simulink library "SHLA_lib"  (Simulink 7.5)
settings: Solver=ode45  StartTime=0.0  StopTime=10.0  RelTol=1e-3
values from neighbouring files (symbols this model uses):
  p_SHLA_LockPVehSpdThd_kmph = Simulink.Parameter    [SHLA_FAW_par.m]
  p_SHLA_SmplCyc_s = Simulink.Parameter    [SHLA_FAW_par.m]
  p_SHLA_TiDlyShiftLvr_s = Simulink.Parameter    [SHLA_FAW_par.m]
  p_SHLA_VehSpdThd_kmph = Simulink.Parameter    [SHLA_FAW_par.m]
  pEpark_st_Parked_C = Simulink.Parameter    [SHLA_FAW_par.m]
  pEpark_st_ParkFlt_C = Simulink.Parameter    [SHLA_FAW_par.m]
  pEpark_st_Parking_C = Simulink.Parameter    [SHLA_FAW_par.m]
  pEpark_st_ParkLocked_C = Simulink.Parameter    [SHLA_FAW_par.m]
  pEpark_st_ParkLockUnknown_C = Simulink.Parameter    [SHLA_FAW_par.m]
  pEpark_st_ParkReq_C = Simulink.Parameter    [SHLA_FAW_par.m]
  pEpark_st_ParkReqOff_C = Simulink.Parameter    [SHLA_FAW_par.m]
  pEpark_st_ParkStalled_C = Simulink.Parameter    [SHLA_FAW_par.m]
  pEpark_st_ParkUnlocked_C = Simulink.Parameter    [SHLA_FAW_par.m]
  pEpark_st_Unparked_C = Simulink.Parameter    [SHLA_FAW_par.m]
  pEpark_st_UnparkedStalled_C = Simulink.Parameter    [SHLA_FAW_par.m]
  pEpark_st_Unparking_C = Simulink.Parameter    [SHLA_FAW_par.m]
  pEpark_st_UnParkReq_C = Simulink.Parameter    [SHLA_FAW_par.m]
  pSHLA_s_StalledDelyTime_C = Simulink.Parameter    [SHLA_FAW_par.m]
undefined symbols (not defined in the file or in its folder): DiscIntNeverNeededParam, p_bool_False_M, p_bool_True_M, pMCI_rpm_VehMoveSpdThrsh_C, pMCI_rpm_VehStdStlSpdThrsh_C, pMCI_s_VehStdStlDly_C, PrkgLockStsTyp, pSHLI_bool_EparkStEnbl, ShiftLvrPosnICTyp, ShiftLvrPosnTyp
libraries: BaseOperationLib_Browser x49, PES_CZ_FAW x2, simulink x2
settings Model: Creator=wuaibin  LastModifiedBy=wuaibin

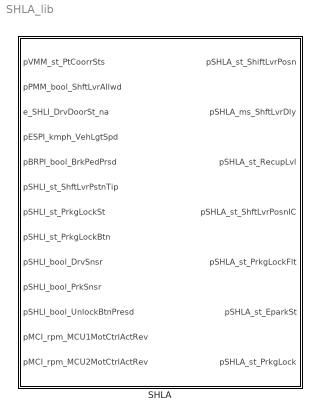
== system SHLA_lib ==
  SHLA : Subsystem  TreatAsAtomicUnit=on

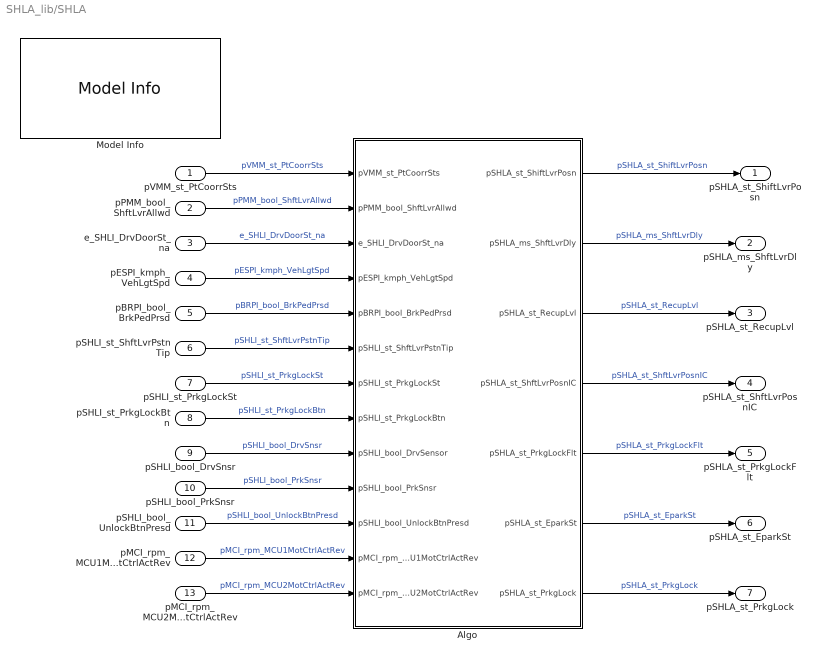
== system SHLA_lib/SHLA ==
  pVMM_st_PtCoorrSts : Inport  OutDataType=fixdt(1, 16)  OutScaling=2^0
  pPMM_bool_ShftLvrAllwd : Inport  Port=2  OutDataType=fixdt(1, 16)  OutScaling=2^0
  e_SHLI_DrvDoorSt_na : Inport  Port=3  OutDataType=fixdt(1, 16)  OutScaling=2^0
  pESPI_kmph_VehLgtSpd : Inport  Port=4  OutDataType=fixdt(1, 16)  OutScaling=2^0
  pBRPI_bool_BrkPedPrsd : Inport  Port=5  OutDataType=fixdt(1, 16)  OutScaling=2^0
  pSHLI_st_ShftLvrPstnTip : Inport  Port=6  OutDataType=fixdt(1, 16)  OutScaling=2^0
  pSHLI_st_PrkgLockSt : Inport  Port=7  OutDataType=fixdt(1, 16)  OutScaling=2^0
  pSHLI_st_PrkgLockBtn : Inport  Port=8  OutDataType=fixdt(1, 16)  OutScaling=2^0
  pSHLI_bool_DrvSnsr : Inport  Port=9
  pSHLI_bool_PrkSnsr : Inport  Port=10
  pSHLI_bool_UnlockBtnPresd : Inport  Port=11
  pMCI_rpm_MCU1MotCtrlActRev : Inport  Port=12
  pMCI_rpm_MCU2MotCtrlActRev : Inport  Port=13
  Algo : Subsystem  TreatAsAtomicUnit=on
  Model Info : simulink/Model-Wide Utilities/Model Info  SystemSampleTime=-1  InitialBlockCM=None  BlockCM=None  Frame=on  DisplayStringWithTags=Model Info\nCreated: %<Created>\nCreator: wuaibin  HorizontalTextAlignment=Center  LeftAlignmentValue=0.5  SourceBlockDiagram=HQEV_HCU  TagMaxNumber=20
  pSHLA_st_ShiftLvrPosn : Outport
  pSHLA_ms_ShftLvrDly : Outport  Port=2
  pSHLA_st_RecupLvl : Outport  Port=3
  pSHLA_st_ShftLvrPosnIC : Outport  Port=4
  pSHLA_st_PrkgLockFlt : Outport  Port=5
  pSHLA_st_EparkSt : Outport  Port=6
  pSHLA_st_PrkgLock : Outport  Port=7
  wires:
  pVMM_st_PtCoorrSts/1 -> Algo/1(pVMM_st_PtCoorrSts)  "pVMM_st_PtCoorrSts"
  pPMM_bool_ShftLvrAllwd/1 -> Algo/2(pPMM_bool_ShftLvrAllwd)  "pPMM_bool_ShftLvrAllwd"
  pBRPI_bool_BrkPedPrsd/1 -> Algo/5(pBRPI_bool_BrkPedPrsd)  "pBRPI_bool_BrkPedPrsd"
  pESPI_kmph_VehLgtSpd/1 -> Algo/4(pESPI_kmph_VehLgtSpd)  "pESPI_kmph_VehLgtSpd"
  pSHLI_st_ShftLvrPstnTip/1 -> Algo/6(pSHLI_st_ShftLvrPstnTip)  "pSHLI_st_ShftLvrPstnTip"
  pSHLI_st_PrkgLockSt/1 -> Algo/7(pSHLI_st_PrkgLockSt)  "pSHLI_st_PrkgLockSt"
  pSHLI_st_PrkgLockBtn/1 -> Algo/8(pSHLI_st_PrkgLockBtn)  "pSHLI_st_PrkgLockBtn"
  pSHLI_bool_DrvSnsr/1 -> Algo/9(pSHLI_bool_DrvSensor)  "pSHLI_bool_DrvSnsr"
  pSHLI_bool_PrkSnsr/1 -> Algo/10(pSHLI_bool_PrkSnsr)  "pSHLI_bool_PrkSnsr"
  Algo/2(pSHLA_ms_ShftLvrDly) -> pSHLA_ms_ShftLvrDly/1  "pSHLA_ms_ShftLvrDly"
  Algo/6(pSHLA_st_EparkSt) -> pSHLA_st_EparkSt/1  "pSHLA_st_EparkSt"
  Algo/3(pSHLA_st_RecupLvl) -> pSHLA_st_RecupLvl/1  "pSHLA_st_RecupLvl"
  Algo/1(pSHLA_st_ShiftLvrPosn) -> pSHLA_st_ShiftLvrPosn/1  "pSHLA_st_ShiftLvrPosn"
  Algo/5(pSHLA_st_PrkgLockFlt) -> pSHLA_st_PrkgLockFlt/1  "pSHLA_st_PrkgLockFlt"
  Algo/4(pSHLA_st_ShftLvrPosnIC) -> pSHLA_st_ShftLvrPosnIC/1  "pSHLA_st_ShftLvrPosnIC"
  Algo/7(pSHLA_st_PrkgLock) -> pSHLA_st_PrkgLock/1  "pSHLA_st_PrkgLock"
  pSHLI_bool_UnlockBtnPresd/1 -> Algo/11(pSHLI_bool_UnlockBtnPresd)  "pSHLI_bool_UnlockBtnPresd"
  pMCI_rpm_MCU1MotCtrlActRev/1 -> Algo/12(pMCI_rpm_MCU1MotCtrlActRev)  "pMCI_rpm_MCU1MotCtrlActRev"
  pMCI_rpm_MCU2MotCtrlActRev/1 -> Algo/13(pMCI_rpm_MCU2MotCtrlActRev)  "pMCI_rpm_MCU2MotCtrlActRev"
  e_SHLI_DrvDoorSt_na/1 -> Algo/3(e_SHLI_DrvDoorSt_na)  "e_SHLI_DrvDoorSt_na"

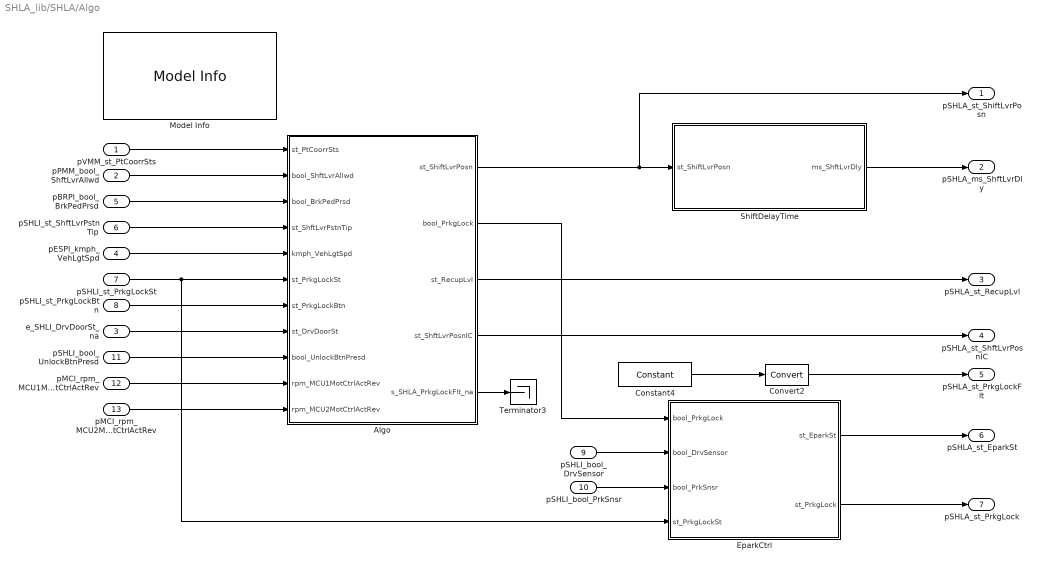
== system SHLA_lib/SHLA/Algo ==
  pVMM_st_PtCoorrSts : Inport  OutDataType=fixdt(1, 16)  OutScaling=2^0
  pPMM_bool_ShftLvrAllwd : Inport  Port=2  OutDataType=fixdt(1, 16)  OutScaling=2^0
  e_SHLI_DrvDoorSt_na : Inport  Port=3  OutDataType=fixdt(1, 16)  OutScaling=2^0
  pESPI_kmph_VehLgtSpd : Inport  Port=4  OutDataType=fixdt(1, 16)  OutScaling=2^0
  pBRPI_bool_BrkPedPrsd : Inport  Port=5  OutDataType=fixdt(1, 16)  OutScaling=2^0
  pSHLI_st_ShftLvrPstnTip : Inport  Port=6  OutDataType=fixdt(1, 16)  OutScaling=2^0
  pSHLI_st_PrkgLockSt : Inport  Port=7  OutDataType=fixdt(1, 16)  OutScaling=2^0
  pSHLI_st_PrkgLockBtn : Inport  Port=8  OutDataType=fixdt(1, 16)  OutScaling=2^0
  pSHLI_bool_DrvSensor : Inport  Port=9
  pSHLI_bool_PrkSnsr : Inport  Port=10
  pSHLI_bool_UnlockBtnPresd : Inport  Port=11  OutDataType=fixdt(1, 16)  OutScaling=2^0
  pMCI_rpm_MCU1MotCtrlActRev : Inport  Port=12
  pMCI_rpm_MCU2MotCtrlActRev : Inport  Port=13
  Algo : Subsystem
  Constant4 : BaseOperationLib_Browser/Sources&Sinks/Constant  Value=p_bool_False_M  OutMin=[]  OutMax=[]  OutDataType=fixdt(1, 16)  ConRadixGroup=Use specified scaling  OutScaling=2^0  OutDataTypeStr=Inherit: Inherit from 'Constant value'
  Convert2 : DataTypeConversion  OutDataType=fixdt(1, 16)  OutScaling=2^0
  EparkCtrl : Subsystem
  Model Info : simulink/Model-Wide Utilities/Model Info  SystemSampleTime=-1  InitialBlockCM=None  BlockCM=None  Frame=on  DisplayStringWithTags=Model Info\nCreated: %<Created>\nCreator: %<Creator>  HorizontalTextAlignment=Center  LeftAlignmentValue=0.5  SourceBlockDiagram=HQEV_HCU  TagMaxNumber=20
  ShiftDelayTime : Subsystem
  Terminator3 : Terminator
  pSHLA_st_ShiftLvrPosn : Outport
  pSHLA_ms_ShftLvrDly : Outport  Port=2
  pSHLA_st_RecupLvl : Outport  Port=3
  pSHLA_st_ShftLvrPosnIC : Outport  Port=4
  pSHLA_st_PrkgLockFlt : Outport  Port=5
  pSHLA_st_EparkSt : Outport  Port=6
  pSHLA_st_PrkgLock : Outport  Port=7
  wires:
  pSHLI_bool_UnlockBtnPresd/1 -> Algo/9(bool_UnlockBtnPresd)
  e_SHLI_DrvDoorSt_na/1 -> Algo/8(st_DrvDoorSt)
  ShiftDelayTime/1(ms_ShftLvrDly) -> pSHLA_ms_ShftLvrDly/1
  pBRPI_bool_BrkPedPrsd/1 -> Algo/3(bool_BrkPedPrsd)
  pSHLI_st_ShftLvrPstnTip/1 -> Algo/4(st_ShftLvrPstnTip)
  pPMM_bool_ShftLvrAllwd/1 -> Algo/2(bool_ShftLvrAllwd)
  pESPI_kmph_VehLgtSpd/1 -> Algo/5(kmph_VehLgtSpd)
  pVMM_st_PtCoorrSts/1 -> Algo/1(st_PtCoorrSts)
  Algo/3(st_RecupLvl) -> pSHLA_st_RecupLvl/1
  pSHLI_st_PrkgLockSt/1 -> EparkCtrl/4(st_PrkgLockSt), Algo/6(st_PrkgLockSt)
  pSHLI_st_PrkgLockBtn/1 -> Algo/7(st_PrkgLockBtn)
  Convert2/1 -> pSHLA_st_PrkgLockFlt/1
  Algo/4(st_ShftLvrPosnIC) -> pSHLA_st_ShftLvrPosnIC/1
  Algo/1(st_ShiftLvrPosn) -> pSHLA_st_ShiftLvrPosn/1, ShiftDelayTime/1(st_ShiftLvrPosn)
  Constant4/1 -> Convert2/1
  Algo/5(s_SHLA_PrkgLockFlt_na) -> Terminator3/1
  pSHLI_bool_DrvSensor/1 -> EparkCtrl/2(bool_DrvSensor)
  pSHLI_bool_PrkSnsr/1 -> EparkCtrl/3(bool_PrkSnsr)
  EparkCtrl/1(st_EparkSt) -> pSHLA_st_EparkSt/1
  Algo/2(bool_PrkgLock) -> EparkCtrl/1(bool_PrkgLock)
  EparkCtrl/2(st_PrkgLock) -> pSHLA_st_PrkgLock/1
  pMCI_rpm_MCU1MotCtrlActRev/1 -> Algo/10(rpm_MCU1MotCtrlActRev)
  pMCI_rpm_MCU2MotCtrlActRev/1 -> Algo/11(rpm_MCU2MotCtrlActRev)

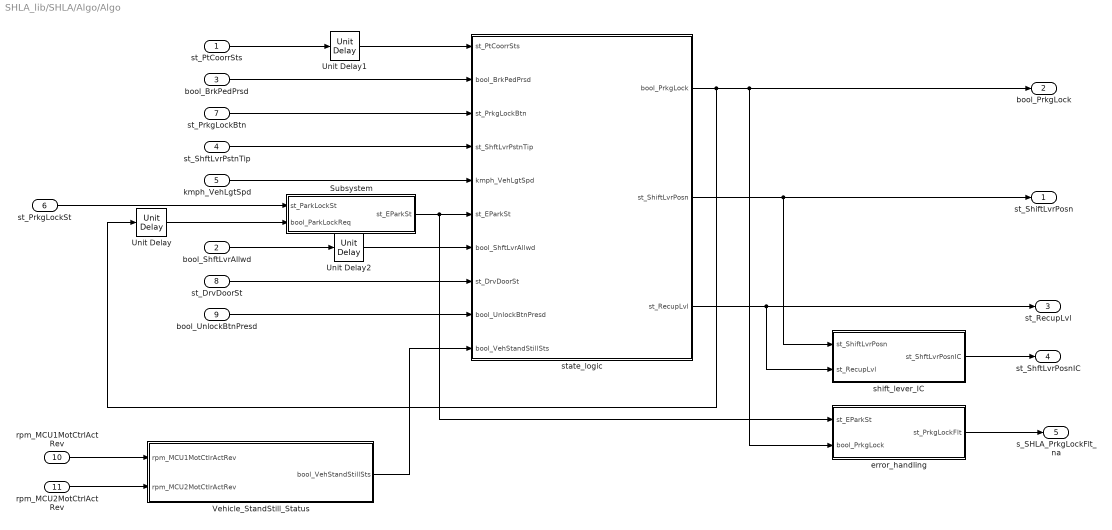
== system SHLA_lib/SHLA/Algo/Algo ==
  st_PtCoorrSts : Inport  OutDataType=fixdt(1, 16)  OutScaling=2^0
  bool_ShftLvrAllwd : Inport  Port=2  OutDataType=fixdt(1, 16)  OutScaling=2^0
  bool_BrkPedPrsd : Inport  Port=3  OutDataType=fixdt(1, 16)  OutScaling=2^0
  st_ShftLvrPstnTip : Inport  Port=4  OutDataType=fixdt(1, 16)  OutScaling=2^0
  kmph_VehLgtSpd : Inport  Port=5  OutDataType=fixdt(1, 16)  OutScaling=2^0
  st_PrkgLockSt : Inport  Port=6  OutDataType=fixdt(1, 16)  OutScaling=2^0
  st_PrkgLockBtn : Inport  Port=7  OutDataType=fixdt(1, 16)  OutScaling=2^0
  st_DrvDoorSt : Inport  Port=8  OutDataType=fixdt(1, 16)  OutScaling=2^0
  bool_UnlockBtnPresd : Inport  Port=9  OutDataType=fixdt(1, 16)  OutScaling=2^0
  rpm_MCU1MotCtrlActRev : Inport  Port=10
  rpm_MCU2MotCtrlActRev : Inport  Port=11
  Subsystem : Subsystem
  Unit Delay : BaseOperationLib_Browser/Discrete Unchanged /Unit Delay  X0=0  SampleTime=-1
  Unit Delay1 : BaseOperationLib_Browser/Discrete Unchanged /Unit Delay  X0=0  SampleTime=-1
  Unit Delay2 : BaseOperationLib_Browser/Discrete Unchanged /Unit Delay  X0=0  SampleTime=-1
  Vehicle_StandStill_Status : Subsystem
  error_handling : Subsystem
  shift_lever_IC : Subsystem
  state_logic : Stateflow chart  TreatAsAtomicUnit=on
  st_ShiftLvrPosn : Outport  OutDataType=fixdt(1, 16)  OutScaling=2^0
  bool_PrkgLock : Outport  Port=2  OutDataType=fixdt(1, 16)  OutScaling=2^0
  st_RecupLvl : Outport  Port=3  OutDataType=fixdt(1, 16)  OutScaling=2^0
  st_ShftLvrPosnIC : Outport  Port=4  OutDataType=fixdt(1, 16)  OutScaling=2^0
  s_SHLA_PrkgLockFlt_na : Outport  Port=5  OutDataType=fixdt(1, 16)  OutScaling=2^0
  wires:
  Unit Delay2/1 -> state_logic/7(bool_ShftLvrAllwd)
  Unit Delay1/1 -> state_logic/1(st_PtCoorrSts)
  bool_UnlockBtnPresd/1 -> state_logic/9(bool_UnlockBtnPresd)
  st_DrvDoorSt/1 -> state_logic/8(st_DrvDoorSt)
  Unit Delay/1 -> Subsystem/2(bool_ParkLockReq)
  st_PrkgLockSt/1 -> Subsystem/1(st_ParkLockSt)
  Subsystem/1(st_EParkSt) -> state_logic/6(st_EParkSt), error_handling/1(st_EParkSt)
  bool_ShftLvrAllwd/1 -> Unit Delay2/1
  error_handling/1(st_PrkgLockFlt) -> s_SHLA_PrkgLockFlt_na/1
  shift_lever_IC/1(st_ShftLvrPosnIC) -> st_ShftLvrPosnIC/1
  st_PtCoorrSts/1 -> Unit Delay1/1
  state_logic/1(bool_PrkgLock) -> Unit Delay/1, bool_PrkgLock/1, error_handling/2(bool_PrkgLock)
  state_logic/2(st_ShiftLvrPosn) -> st_ShiftLvrPosn/1, shift_lever_IC/1(st_ShiftLvrPosn)
  kmph_VehLgtSpd/1 -> state_logic/5(kmph_VehLgtSpd)
  st_ShftLvrPstnTip/1 -> state_logic/4(st_ShftLvrPstnTip)
  bool_BrkPedPrsd/1 -> state_logic/2(bool_BrkPedPrsd)
  state_logic/3(st_RecupLvl) -> st_RecupLvl/1, shift_lever_IC/2(st_RecupLvl)
  st_PrkgLockBtn/1 -> state_logic/3(st_PrkgLockBtn)
  Vehicle_StandStill_Status/1(bool_VehStandStillSts) -> state_logic/10(bool_VehStandStillSts)
  rpm_MCU1MotCtrlActRev/1 -> Vehicle_StandStill_Status/1(rpm_MCU1MotCtlrActRev)
  rpm_MCU2MotCtrlActRev/1 -> Vehicle_StandStill_Status/2(rpm_MCU2MotCtlrActRev)

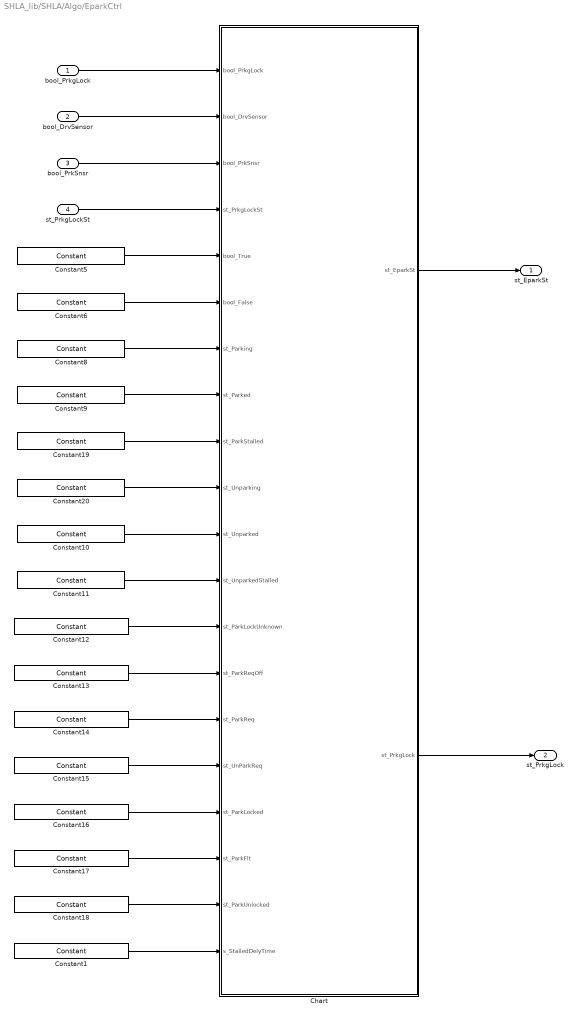
== system SHLA_lib/SHLA/Algo/EparkCtrl ==
  bool_PrkgLock : Inport
  bool_DrvSensor : Inport  Port=2
  bool_PrkSnsr : Inport  Port=3
  st_PrkgLockSt : Inport  Port=4
  Chart : Stateflow chart  TreatAsAtomicUnit=on
  Constant1 : BaseOperationLib_Browser/Sources&Sinks/Constant  Value=pSHLA_s_StalledDelyTime_C  OutMin=[]  OutMax=[]  OutDataType=fixdt(1, 16)  ConRadixGroup=Use specified scaling  OutScaling=2^0  OutDataTypeStr=Inherit: Inherit from 'Constant value'
  Constant10 : BaseOperationLib_Browser/Sources&Sinks/Constant  Value=pEpark_st_Unparked_C  OutMin=[]  OutMax=[]  OutDataType=fixdt(1, 16)  ConRadixGroup=Use specified scaling  OutScaling=2^0  OutDataTypeStr=Inherit: Inherit from 'Constant value'
  Constant11 : BaseOperationLib_Browser/Sources&Sinks/Constant  Value=pEpark_st_UnparkedStalled_C  OutMin=[]  OutMax=[]  OutDataType=fixdt(1, 16)  ConRadixGroup=Use specified scaling  OutScaling=2^0  OutDataTypeStr=Inherit: Inherit from 'Constant value'
  Constant12 : BaseOperationLib_Browser/Sources&Sinks/Constant  Value=pEpark_st_ParkLockUnknown_C  OutMin=[]  OutMax=[]  OutDataType=fixdt(1, 16)  ConRadixGroup=Use specified scaling  OutScaling=2^0  OutDataTypeStr=Inherit: Inherit from 'Constant value'
  Constant13 : BaseOperationLib_Browser/Sources&Sinks/Constant  Value=pEpark_st_ParkReqOff_C  OutMin=[]  OutMax=[]  OutDataType=fixdt(1, 16)  ConRadixGroup=Use specified scaling  OutScaling=2^0  OutDataTypeStr=Inherit: Inherit from 'Constant value'
  Constant14 : BaseOperationLib_Browser/Sources&Sinks/Constant  Value=pEpark_st_ParkReq_C  OutMin=[]  OutMax=[]  OutDataType=fixdt(1, 16)  ConRadixGroup=Use specified scaling  OutScaling=2^0  OutDataTypeStr=Inherit: Inherit from 'Constant value'
  Constant15 : BaseOperationLib_Browser/Sources&Sinks/Constant  Value=pEpark_st_UnParkReq_C  OutMin=[]  OutMax=[]  OutDataType=fixdt(1, 16)  ConRadixGroup=Use specified scaling  OutScaling=2^0  OutDataTypeStr=Inherit: Inherit from 'Constant value'
  Constant16 : BaseOperationLib_Browser/Sources&Sinks/Constant  Value=pEpark_st_ParkLocked_C  OutMin=[]  OutMax=[]  OutDataType=fixdt(1, 16)  ConRadixGroup=Use specified scaling  OutScaling=2^0  OutDataTypeStr=Inherit: Inherit from 'Constant value'
  Constant17 : BaseOperationLib_Browser/Sources&Sinks/Constant  Value=pEpark_st_ParkFlt_C  OutMin=[]  OutMax=[]  OutDataType=fixdt(1, 16)  ConRadixGroup=Use specified scaling  OutScaling=2^0  OutDataTypeStr=Inherit: Inherit from 'Constant value'
  Constant18 : BaseOperationLib_Browser/Sources&Sinks/Constant  Value=pEpark_st_ParkUnlocked_C  OutMin=[]  OutMax=[]  OutDataType=fixdt(1, 16)  ConRadixGroup=Use specified scaling  OutScaling=2^0  OutDataTypeStr=Inherit: Inherit from 'Constant value'
  Constant19 : BaseOperationLib_Browser/Sources&Sinks/Constant  Value=pEpark_st_ParkStalled_C  OutMin=[]  OutMax=[]  OutDataType=fixdt(1, 16)  ConRadixGroup=Use specified scaling  OutScaling=2^0  OutDataTypeStr=Inherit: Inherit from 'Constant value'
  Constant20 : BaseOperationLib_Browser/Sources&Sinks/Constant  Value=pEpark_st_Unparking_C  OutMin=[]  OutMax=[]  OutDataType=fixdt(1, 16)  ConRadixGroup=Use specified scaling  OutScaling=2^0  OutDataTypeStr=Inherit: Inherit from 'Constant value'
  Constant5 : BaseOperationLib_Browser/Sources&Sinks/Constant  Value=p_bool_True_M  OutMin=[]  OutMax=[]  OutDataType=fixdt(1, 16)  ConRadixGroup=Use specified scaling  OutScaling=2^0  OutDataTypeStr=Inherit: Inherit from 'Constant value'
  Constant6 : BaseOperationLib_Browser/Sources&Sinks/Constant  Value=p_bool_False_M  OutMin=[]  OutMax=[]  OutDataType=fixdt(1, 16)  ConRadixGroup=Use specified scaling  OutScaling=2^0  OutDataTypeStr=Inherit: Inherit from 'Constant value'
  Constant8 : BaseOperationLib_Browser/Sources&Sinks/Constant  Value=pEpark_st_Parking_C  OutMin=[]  OutMax=[]  OutDataType=fixdt(1, 16)  ConRadixGroup=Use specified scaling  OutScaling=2^0  OutDataTypeStr=Inherit: Inherit from 'Constant value'
  Constant9 : BaseOperationLib_Browser/Sources&Sinks/Constant  Value=pEpark_st_Parked_C  OutMin=[]  OutMax=[]  OutDataType=fixdt(1, 16)  ConRadixGroup=Use specified scaling  OutScaling=2^0  OutDataTypeStr=Inherit: Inherit from 'Constant value'
  st_EparkSt : Outport
  st_PrkgLock : Outport  Port=2
  wires:
  Constant1/1 -> Chart/20(s_StalledDelyTime)
  bool_DrvSensor/1 -> Chart/2(bool_DrvSensor)
  bool_PrkSnsr/1 -> Chart/3(bool_PrkSnsr)
  Chart/1(st_EparkSt) -> st_EparkSt/1
  Constant5/1 -> Chart/5(bool_True)
  Constant6/1 -> Chart/6(bool_False)
  Constant8/1 -> Chart/7(st_Parking)
  Constant9/1 -> Chart/8(st_Parked)
  Constant19/1 -> Chart/9(st_ParkStalled)
  Constant20/1 -> Chart/10(st_Unparking)
  Constant10/1 -> Chart/11(st_Unparked)
  Constant11/1 -> Chart/12(st_UnparkedStalled)
  Constant12/1 -> Chart/13(st_ParkLockUnknown)
  Constant13/1 -> Chart/14(st_ParkReqOff)
  Constant14/1 -> Chart/15(st_ParkReq)
  Constant15/1 -> Chart/16(st_UnParkReq)
  Constant16/1 -> Chart/17(st_ParkLocked)
  Constant17/1 -> Chart/18(st_ParkFlt)
  Constant18/1 -> Chart/19(st_ParkUnlocked)
  bool_PrkgLock/1 -> Chart/1(bool_PrkgLock)
  st_PrkgLockSt/1 -> Chart/4(st_PrkgLockSt)
  Chart/2(st_PrkgLock) -> st_PrkgLock/1

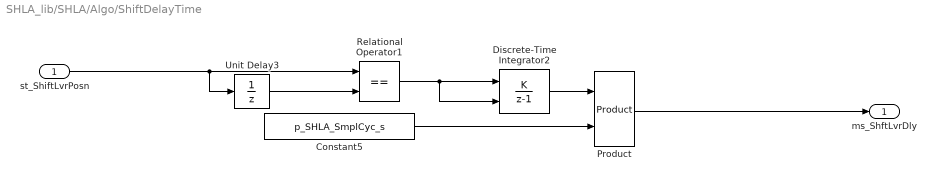
== system SHLA_lib/SHLA/Algo/ShiftDelayTime ==
  st_ShiftLvrPosn : Inport  PortDimensions=1  OutDataType=fixdt(1, 16)  OutScaling=2^0
  Constant5 : Constant  Value=p_SHLA_SmplCyc_s  OutDataType=Enum: ShiftLvrPosnICTyp  ConRadixGroup=Best Precision: Vector-wise
      mask Display: patch([0 1 1 1 .75], [1 1 0 .75 1], [0 1 0]);
  Discrete-Time Integrator2 : DiscreteIntegrator  IntegratorMethod=Accumulation: Forward Euler  ExternalReset=falling  SampleTime=-1  OutDataType=PDT_s  OutDataTypeStr=Inherit: Inherit via back propagation  LimitOutput=on  UpperSaturationLimit=200  LowerSaturationLimit=0  ICPrevOutput=DiscIntNeverNeededParam  ICPrevScaledInput=DiscIntNeverNeededParam
  Product : BaseOperationLib_Browser/Math Operations Changed/Product  Inputs=2  Multiplication=Element-wise(.*)  OutMin=[]  OutMax=[]  OutDataType=fixdt(1,16,0)  OutScaling=[]  OutDataTypeStr=Inherit: Inherit via back propagation  RndMeth=Zero  SaturateOnIntegerOverflow=on
  Relational Operator1 : RelationalOperator  Operator===  LogicOutDataTypeMode=boolean  OutDataTypeStr=boolean
  Unit Delay3 : UnitDelay  SampleTime=-1
  ms_ShftLvrDly : Outport  PortDimensions=1  OutDataType=fixdt(1, 16)  OutScaling=2^0
  wires:
  st_ShiftLvrPosn/1 -> Unit Delay3/1, Relational Operator1/1
  Relational Operator1/1 -> Discrete-Time Integrator2/1, Discrete-Time Integrator2/2
  Unit Delay3/1 -> Relational Operator1/2
  Discrete-Time Integrator2/1 -> Product/1
  Constant5/1 -> Product/2
  Product/1 -> ms_ShftLvrDly/1

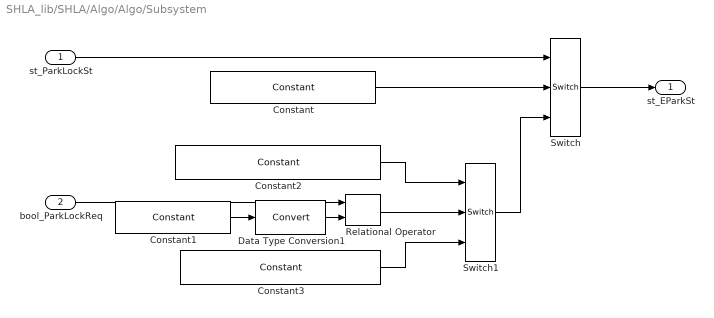
== system SHLA_lib/SHLA/Algo/Algo/Subsystem ==
  st_ParkLockSt : Inport  OutDataType=fixdt(1, 16)  OutScaling=2^0
  bool_ParkLockReq : Inport  Port=2  OutDataType=fixdt(1, 16)  OutScaling=2^0
  Constant : BaseOperationLib_Browser/Sources&Sinks/Constant  Value=pSHLI_bool_EparkStEnbl  OutMin=[]  OutMax=[]  OutDataType=fixdt(1, 16)  ConRadixGroup=Use specified scaling  OutScaling=2^0  OutDataTypeStr=Inherit: Inherit from 'Constant value'
  Constant1 : BaseOperationLib_Browser/Sources&Sinks/Constant  Value=p_bool_True_M  OutMin=[]  OutMax=[]  OutDataType=fixdt(1, 16)  ConRadixGroup=Use specified scaling  OutScaling=2^0  OutDataTypeStr=Inherit: Inherit from 'Constant value'
  Constant2 : BaseOperationLib_Browser/Sources&Sinks/Constant  Value=uint8(PrkgLockStsTyp.PLS_PARKED)  OutMin=[]  OutMax=[]  OutDataType=Enum: PrkgLockStsTyp  ConRadixGroup=Best Precision: Vector-wise  OutScaling=[]  OutDataTypeStr=Inherit: Inherit from 'Constant value'
  Constant3 : BaseOperationLib_Browser/Sources&Sinks/Constant  Value=uint8(PrkgLockStsTyp.PLS_UNPARKED)  OutMin=[]  OutMax=[]  OutDataType=Enum: PrkgLockStsTyp  ConRadixGroup=Best Precision: Vector-wise  OutScaling=[]  OutDataTypeStr=Inherit: Inherit from 'Constant value'
  Data Type Conversion1 : DataTypeConversion  OutDataType=fixdt(1, 16)  OutScaling=2^0
  Relational Operator : BaseOperationLib_Browser/Logic Operations Changed/Relational Operator  Operator===  InputSameDT=on  LogicOutDataTypeMode=Specify via dialog  LogicDataType=PDT_Bool  OutDataTypeStr=PDT_Bool
  Switch : BaseOperationLib_Browser/Signal Routing Changed/Switch  Criteria=u2 ~= 0  Threshold=1  InputSameDT=on  OutMin=[]  OutMax=[]  OutDataType=fixdt(1,16,0)  OutScaling=[]  SaturateOnIntegerOverflow=on
  Switch1 : BaseOperationLib_Browser/Signal Routing Changed/Switch  Criteria=u2 ~= 0  Threshold=1  InputSameDT=on  OutMin=[]  OutMax=[]  OutDataType=fixdt(1,16,0)  OutScaling=[]  SaturateOnIntegerOverflow=on
  st_EParkSt : Outport  OutDataType=fixdt(1, 16)  OutScaling=2^0
  wires:
  Data Type Conversion1/1 -> Relational Operator/2
  Constant2/1 -> Switch1/1
  Switch1/1 -> Switch/3
  Constant1/1 -> Data Type Conversion1/1
  Relational Operator/1 -> Switch1/2
  bool_ParkLockReq/1 -> Relational Operator/1
  Switch/1 -> st_EParkSt/1
  st_ParkLockSt/1 -> Switch/1
  Constant/1 -> Switch/2
  Constant3/1 -> Switch1/3

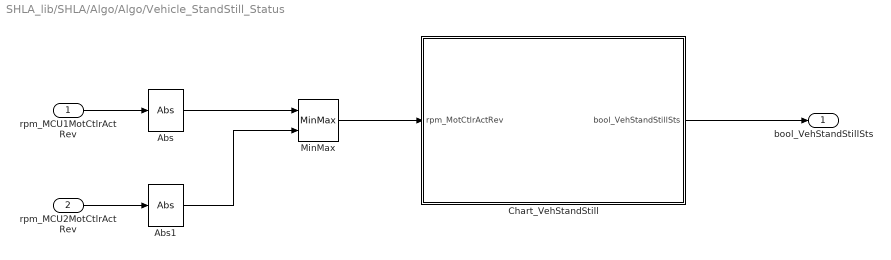
== system SHLA_lib/SHLA/Algo/Algo/Vehicle_StandStill_Status ==
  rpm_MCU1MotCtlrActRev : Inport  OutDataType=fixdt(1, 16)  OutScaling=2^0
  rpm_MCU2MotCtlrActRev : Inport  Port=2  OutDataType=fixdt(1, 16)  OutScaling=2^0
  Abs : BaseOperationLib_Browser/Math Operations Changed/Abs  OutMax=[]  OutDataType=fixdt(1, 16)  OutScaling=2^0  SaturateOnIntegerOverflow=on
  Abs1 : BaseOperationLib_Browser/Math Operations Changed/Abs  OutMax=[]  OutDataType=fixdt(1, 16)  OutScaling=2^0  SaturateOnIntegerOverflow=on
  Chart_VehStandStill : Stateflow chart  TreatAsAtomicUnit=on
  MinMax : BaseOperationLib_Browser/Math Operations Changed/MinMax  Function=max  Inputs=2  InputSameDT=on  OutMin=[]  OutMax=[]  OutDataType=fixdt(1, 16)  OutScaling=2^0  SaturateOnIntegerOverflow=on
  bool_VehStandStillSts : Outport
  wires:
  rpm_MCU1MotCtlrActRev/1 -> Abs/1
  Chart_VehStandStill/1(bool_VehStandStillSts) -> bool_VehStandStillSts/1
  rpm_MCU2MotCtlrActRev/1 -> Abs1/1
  MinMax/1 -> Chart_VehStandStill/1(rpm_MotCtlrActRev)
  Abs/1 -> MinMax/1
  Abs1/1 -> MinMax/2

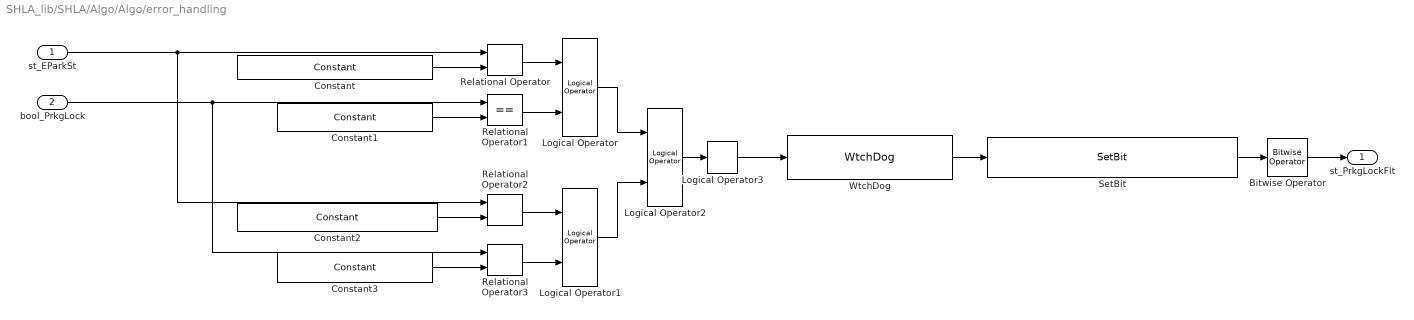
== system SHLA_lib/SHLA/Algo/Algo/error_handling ==
  st_EParkSt : Inport
  bool_PrkgLock : Inport  Port=2
  Bitwise Operator : BaseOperationLib_Browser/Others Unchanged/Bitwise Operator  logicop=OR  UseBitMask=off  BitMask=bin2dec('11011001')  BitMaskRealWorld=Stored Integer
  Constant : BaseOperationLib_Browser/Sources&Sinks/Constant  Value=uint8(PrkgLockStsTyp.PLS_PARKED)  OutMin=[]  OutMax=[]  OutDataType=Enum: PrkgLockStsTyp  ConRadixGroup=Best Precision: Vector-wise  OutScaling=[]  OutDataTypeStr=Inherit: Inherit from 'Constant value'
  Constant1 : BaseOperationLib_Browser/Sources&Sinks/Constant  Value=p_bool_True_M  OutMin=[]  OutMax=[]  OutDataType=Enum: ShiftLvrPosnTyp  ConRadixGroup=Best Precision: Vector-wise  OutScaling=[]  OutDataTypeStr=Inherit: Inherit via back propagation
  Constant2 : BaseOperationLib_Browser/Sources&Sinks/Constant  Value=uint8(PrkgLockStsTyp.PLS_UNPARKED)  OutMin=[]  OutMax=[]  OutDataType=Enum: PrkgLockStsTyp  ConRadixGroup=Best Precision: Vector-wise  OutScaling=[]  OutDataTypeStr=Inherit: Inherit from 'Constant value'
  Constant3 : BaseOperationLib_Browser/Sources&Sinks/Constant  Value=p_bool_False_M  OutMin=[]  OutMax=[]  OutDataType=Enum: ShiftLvrPosnTyp  ConRadixGroup=Best Precision: Vector-wise  OutScaling=[]  OutDataTypeStr=Inherit: Inherit from 'Constant value'
  Logical Operator : BaseOperationLib_Browser/Logic Operations Changed/Logical Operator  Operator=AND  Inputs=2  AllPortsSameDT=on  OutDataTypeMode=Specify via dialog  LogicDataType=PDT_Bool  OutDataTypeStr=PDT_Bool
  Logical Operator1 : BaseOperationLib_Browser/Logic Operations Changed/Logical Operator  Operator=AND  Inputs=2  AllPortsSameDT=on  OutDataTypeMode=Specify via dialog  LogicDataType=PDT_Bool  OutDataTypeStr=PDT_Bool
  Logical Operator2 : BaseOperationLib_Browser/Logic Operations Changed/Logical Operator  Operator=OR  Inputs=2  AllPortsSameDT=on  OutDataTypeMode=Specify via dialog  LogicDataType=PDT_Bool  OutDataTypeStr=PDT_Bool
  Logical Operator3 : BaseOperationLib_Browser/Logic Operations Changed/Logical Operator  Operator=NOT  Inputs=2  AllPortsSameDT=on  OutDataTypeMode=Specify via dialog  LogicDataType=PDT_Bool  OutDataTypeStr=PDT_Bool
  Relational Operator : BaseOperationLib_Browser/Logic Operations Changed/Relational Operator  Operator=~=  InputSameDT=on  LogicOutDataTypeMode=Specify via dialog  LogicDataType=PDT_Bool  OutDataTypeStr=PDT_Bool
  Relational Operator1 : RelationalOperator  Operator===  LogicOutDataTypeMode=Specify via dialog  LogicDataType=PDT_Bool  OutDataTypeStr=PDT_Bool  InputSameDT=on
      mask Display: patch([0 1 1 1 .75], [1 1 0 .75 1], [0 1 0]);
  Relational Operator2 : BaseOperationLib_Browser/Logic Operations Changed/Relational Operator  Operator=~=  InputSameDT=on  LogicOutDataTypeMode=Specify via dialog  LogicDataType=PDT_Bool  OutDataTypeStr=PDT_Bool
  Relational Operator3 : BaseOperationLib_Browser/Logic Operations Changed/Relational Operator  Operator===  InputSameDT=on  LogicOutDataTypeMode=Specify via dialog  LogicDataType=PDT_Bool  OutDataTypeStr=PDT_Bool
  SetBit : PES_CZ_FAW/Discontinuities/SetBit  SystemSampleTime=-1  maska=PrkgLockFltTyp.E_PARK_PLAUSIBILITY_ERR
  WtchDog : PES_CZ_FAW/Discontinuities/WtchDog  SystemSampleTime=-1  timeoutthres=p_SHLA_TiDlyPrkLock_s
  st_PrkgLockFlt : Outport
  wires:
  WtchDog/1 -> SetBit/1
  bool_PrkgLock/1 -> Relational Operator1/1, Relational Operator3/1
  st_EParkSt/1 -> Relational Operator2/1, Relational Operator/1
  Logical Operator2/1 -> Logical Operator3/1
  Logical Operator1/1 -> Logical Operator2/2
  Logical Operator/1 -> Logical Operator2/1
  Relational Operator3/1 -> Logical Operator1/2
  Relational Operator2/1 -> Logical Operator1/1
  Constant3/1 -> Relational Operator3/2
  Constant2/1 -> Relational Operator2/2
  Relational Operator1/1 -> Logical Operator/2
  Relational Operator/1 -> Logical Operator/1
  Constant1/1 -> Relational Operator1/2
  Constant/1 -> Relational Operator/2
  SetBit/1 -> Bitwise Operator/1
  Bitwise Operator/1 -> st_PrkgLockFlt/1
  Logical Operator3/1 -> WtchDog/1

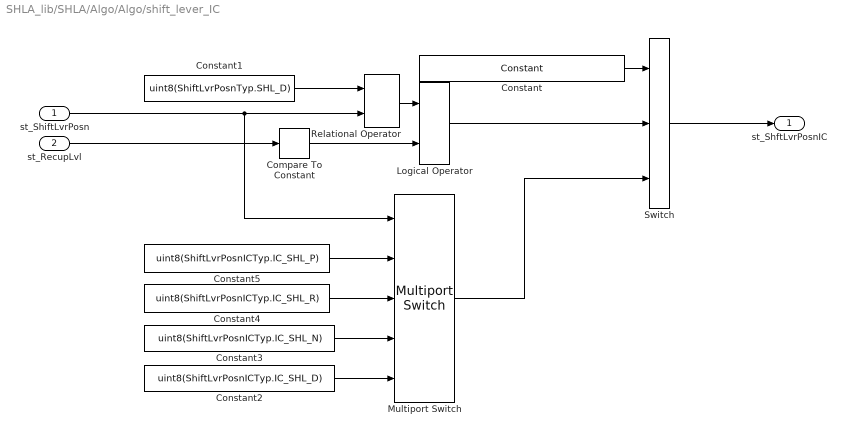
== system SHLA_lib/SHLA/Algo/Algo/shift_lever_IC ==
  st_ShiftLvrPosn : Inport
  st_RecupLvl : Inport  Port=2
  Compare To Constant : BaseOperationLib_Browser/Logic Operations Changed/Compare To Constant  SystemSampleTime=-1  relop=>=  const=true
  Constant : BaseOperationLib_Browser/Sources&Sinks/Constant  Value=uint8(ShiftLvrPosnICTyp.IC_SHL_B)  OutMin=[]  OutMax=[]  OutDataType=Enum: ShiftLvrPosnICTyp  ConRadixGroup=Best Precision: Vector-wise  OutScaling=[]  OutDataTypeStr=Inherit: Inherit from 'Constant value'
  Constant1 : Constant  Value=uint8(ShiftLvrPosnTyp.SHL_D)  OutDataType=Enum: ShiftLvrPosnTyp  ConRadixGroup=Best Precision: Vector-wise
      mask Display: patch([0 1 1 1 .75], [1 1 0 .75 1], [0 1 0]);
  Constant2 : Constant  Value=uint8(ShiftLvrPosnICTyp.IC_SHL_D)  OutDataType=Enum: ShiftLvrPosnICTyp  ConRadixGroup=Best Precision: Vector-wise
      mask Display: patch([0 1 1 1 .75], [1 1 0 .75 1], [0 1 0]);
  Constant3 : Constant  Value=uint8(ShiftLvrPosnICTyp.IC_SHL_N)  OutDataType=Enum: ShiftLvrPosnICTyp  ConRadixGroup=Best Precision: Vector-wise
      mask Display: patch([0 1 1 1 .75], [1 1 0 .75 1], [0 1 0]);
  Constant4 : Constant  Value=uint8(ShiftLvrPosnICTyp.IC_SHL_R)  OutDataType=Enum: ShiftLvrPosnICTyp  ConRadixGroup=Best Precision: Vector-wise
      mask Display: patch([0 1 1 1 .75], [1 1 0 .75 1], [0 1 0]);
  Constant5 : Constant  Value=uint8(ShiftLvrPosnICTyp.IC_SHL_P)  OutDataType=Enum: ShiftLvrPosnICTyp  ConRadixGroup=Best Precision: Vector-wise
      mask Display: patch([0 1 1 1 .75], [1 1 0 .75 1], [0 1 0]);
  Logical Operator : BaseOperationLib_Browser/Logic Operations Changed/Logical Operator  Operator=AND  Inputs=2  AllPortsSameDT=on  OutDataTypeMode=Specify via dialog  LogicDataType=PDT_Bool  OutDataTypeStr=PDT_Bool
  Multiport Switch : BaseOperationLib_Browser/Signal Routing Changed/Multiport Switch  DataPortOrder=Specify indices  Inputs=4  DataPortIndices={uint8(ShiftLvrPosnTyp.SHL_P),uint8(ShiftLvrPosnTyp.SHL_R),uint8(ShiftLvrPosnTyp.SHL_N),uint8(ShiftLvrPosnTyp.SHL_D)}  zeroidx=off  InputSameDT=on  OutMin=[]  OutMax=[]  OutDataType=fixdt(1, 16)  OutScaling=2^0  OutDataTypeStr=Inherit: Inherit via back propagation  SaturateOnIntegerOverflow=on
  Relational Operator : BaseOperationLib_Browser/Logic Operations Changed/Relational Operator  Operator===  InputSameDT=on  LogicOutDataTypeMode=Specify via dialog  LogicDataType=PDT_Bool  OutDataTypeStr=PDT_Bool
  Switch : BaseOperationLib_Browser/Signal Routing Changed/Switch  Criteria=u2 ~= 0  Threshold=1  InputSameDT=on  OutMin=[]  OutMax=[]  OutDataType=fixdt(1,16,0)  OutScaling=[]  SaturateOnIntegerOverflow=on
  st_ShftLvrPosnIC : Outport
  wires:
  Multiport Switch/1 -> Switch/3
  Constant2/1 -> Multiport Switch/5
  Constant3/1 -> Multiport Switch/4
  Constant4/1 -> Multiport Switch/3
  Constant5/1 -> Multiport Switch/2
  Switch/1 -> st_ShftLvrPosnIC/1
  st_RecupLvl/1 -> Compare To Constant/1
  st_ShiftLvrPosn/1 -> Multiport Switch/1, Relational Operator/2
  Constant1/1 -> Relational Operator/1
  Relational Operator/1 -> Logical Operator/1
  Logical Operator/1 -> Switch/2
  Compare To Constant/1 -> Logical Operator/2
  Constant/1 -> Switch/1

== stateflow chart SHLA/Algo/Algo/state_logic ==
  state E_park
    en:
    bool_PrkgLock = true;
    st_RecupLvl = 0;
    state P_LOCK_LOGIC
      state Unparked
        du:
        st_ShiftLvrPosn = ShiftLvrPosnTyp.SHL_N;
      state Parked
        du:
        st_ShiftLvrPosn = ShiftLvrPosnTyp.SHL_P;
      (default) -> Parked
      Parked -> Unparked : [st_EParkSt == PrkgLockStsTyp.PLS_UNPARKED]
      Unparked -> Parked : [st_EParkSt == PrkgLockStsTyp.PLS_PARKED]
  state Drive_ready
    state DRIVE_READY
      state E_park_active
        en:
        bool_PrkgLock = true;
        Drive_ready.DRIVE_READY.E_park_active -> Drive_ready.DRIVE_READY.E_park_active [order 1] : [st_EParkSt == PrkgLockStsTyp.PLS_PARKED && ...
            | st_ShiftLvrPosn ~= ShiftLvrPosnTyp.SHL_P]
            | {st_ShiftLvrPosn = ShiftLvrPosnTyp.SHL_P;}
      state Neutral
        en:
        bool_PrkgLock = false;
        Drive_ready.DRIVE_READY.Neutral -> Drive_ready.DRIVE_READY.Neutral [order 1] : [st_EParkSt == PrkgLockStsTyp.PLS_UNPARKED && ...
            | st_ShiftLvrPosn ~= ShiftLvrPosnTyp.SHL_N]
            | {st_ShiftLvrPosn = ShiftLvrPosnTyp.SHL_N;}
      state Init
      (default) -> Drive_ready.DRIVE_READY.Init
      Drive_ready.DRIVE_READY.Neutral -> Drive_ready.DRIVE_READY.E_park_active [order 1] : [((st_PrkgLockBtn && ...
          | (abs(kmph_VehLgtSpd) < p_SHLA_LockPVehSpdThd_kmph)) || ...
          | (st_DrvDoorSt && ...
          | bool_BrkPedPrsd == false && ...
          | abs(kmph_VehLgtSpd) < p_SHLA_LockPVehSpdThd_kmph)) && ...
          | st_ShiftLvrPosn == ShiftLvrPosnTyp.SHL_N && ...
          | bool_ShftLvrAllwd]
      Drive_ready.DRIVE_READY.E_park_active -> Drive_ready.DRIVE_READY.Neutral [order 1] : [bool_BrkPedPrsd && ...
          | (st_ShftLvrPstnTip == ShiftLvrPosnTipTyp.TIP_UP || ...
          | st_ShftLvrPstnTip == ShiftLvrPosnTipTyp.TIP_DOWN) && ...
          | st_ShiftLvrPosn == ShiftLvrPosnTyp.SHL_P]
      Drive_ready.DRIVE_READY.Init -> Drive_ready.DRIVE_READY.Neutral [order 1] : [st_ShiftLvrPosn == ShiftLvrPosnTyp.SHL_N]
      Drive_ready.DRIVE_READY.Init -> Drive_ready.DRIVE_READY.E_park_active [order 2] : [st_ShiftLvrPosn == ShiftLvrPosnTyp.SHL_P]
  state Driving
    state DRIVING
      state E_park_active
        en:
        bool_PrkgLock = true;
        st_RecupLvl = 0;
        Driving.DRIVING.E_park_active -> Driving.DRIVING.E_park_active [order 1] : [st_EParkSt == PrkgLockStsTyp.PLS_PARKED && ...
            | st_ShiftLvrPosn ~= ShiftLvrPosnTyp.SHL_P]
            | {st_ShiftLvrPosn = ShiftLvrPosnTyp.SHL_P;}
      state E_park_deactive
        en:
        bool_PrkgLock = false;
        state Shift_lever_logic
          state Reverse
            Reverse -> Reverse [order 1] : [st_EParkSt == PrkgLockStsTyp.PLS_UNPARKED && ...
                | st_ShiftLvrPosn ~= ShiftLvrPosnTyp.SHL_R]
                | {st_ShiftLvrPosn = ShiftLvrPosnTyp.SHL_R;
                | st_RecupLvl = 0;}
          state Drive
            state Recuperation
              state No_recuperation
                en:
                st_RecupLvl = 0;
                TranEna = false;
                No_recuperation -> No_recuperation [order 1] : [st_ShftLvrPstnTip == ShiftLvrPosnTipTyp.NO_TIP]
                    | {TranEna = true;}
              state Recuperation
                en:
                st_RecupLvl = 1;
                TranEna = false;
                Driving.DRIVING.E_park_deactive.Shift_lever_logic.Drive.Recuperation.Recuperation -> Driving.DRIVING.E_park_deactive.Shift_lever_logic.Drive.Recuperation.Recuperation [order 1] : [st_ShftLvrPstnTip == ShiftLvrPosnTipTyp.NO_TIP]
                    | {TranEna = true;}
              state Init
                Driving.DRIVING.E_park_deactive.Shift_lever_logic.Drive.Recuperation.Init -> Driving.DRIVING.E_park_deactive.Shift_lever_logic.Drive.Recuperation.Init [order 1] : [st_EParkSt == PrkgLockStsTyp.PLS_UNPARKED && ...
                    | st_ShiftLvrPosn ~= ShiftLvrPosnTyp.SHL_D]
                    | {st_ShiftLvrPosn = ShiftLvrPosnTyp.SHL_D;}
              Driving.DRIVING.E_park_deactive.Shift_lever_logic.Drive.Recuperation.Init -> No_recuperation [order 1] : [st_ShiftLvrPosn == ShiftLvrPosnTyp.SHL_D]
              Driving.DRIVING.E_park_deactive.Shift_lever_logic.Drive.Recuperation.Recuperation -> No_recuperation [order 1] : [st_ShftLvrPstnTip == ShiftLvrPosnTipTyp.TIP_DOWN && ...
                  | TranEna]
              No_recuperation -> Driving.DRIVING.E_park_deactive.Shift_lever_logic.Drive.Recuperation.Recuperation [order 1] : [st_ShftLvrPstnTip == ShiftLvrPosnTipTyp.TIP_DOWN && ...
                  | TranEna]
              (default) -> Driving.DRIVING.E_park_deactive.Shift_lever_logic.Drive.Recuperation.Init
          state Neutral_tmp
          state Neutral
            Driving.DRIVING.E_park_deactive.Shift_lever_logic.Neutral -> Driving.DRIVING.E_park_deactive.Shift_lever_logic.Neutral [order 1] : [st_EParkSt == PrkgLockStsTyp.PLS_UNPARKED && ...
                | st_ShiftLvrPosn ~= ShiftLvrPosnTyp.SHL_N]
                | {st_ShiftLvrPosn = ShiftLvrPosnTyp.SHL_N;
                | st_RecupLvl = 0;}
          (junction 27) -> Reverse [order 2] : [st_ShftLvrPstnTip == ShiftLvrPosnTipTyp.TIP_UP && ...
              | bool_UnlockBtnPresd == true]
          Neutral_tmp -> Driving.DRIVING.E_park_deactive.Shift_lever_logic.Neutral [order 2] : [st_ShftLvrPstnTip == ShiftLvrPosnTipTyp.NO_TIP]
          Driving.DRIVING.E_park_deactive.Shift_lever_logic.Neutral -> Reverse [order 1] : [st_ShftLvrPstnTip == ShiftLvrPosnTipTyp.TIP_UP && ...
              | st_ShiftLvrPosn == ShiftLvrPosnTyp.SHL_N && ...
              | bool_UnlockBtnPresd == true && ...
              | ((bool_VehStandStillSts == true && ...
              | bool_BrkPedPrsd)||...
              | ((bool_VehStandStillSts == false) && ...
              | (kmph_VehLgtSpd < p_SHLA_VehSpdThd_kmph))) && ...
              | bool_ShftLvrAllwd]
          Driving.DRIVING.E_park_deactive.Shift_lever_logic.Neutral -> Drive [order 2] : [st_ShftLvrPstnTip == ShiftLvrPosnTipTyp.TIP_DOWN && ...
              | st_ShiftLvrPosn == ShiftLvrPosnTyp.SHL_N&& ...
              | ((bool_VehStandStillSts == true && ...
              | bool_BrkPedPrsd) || ...
              | ((bool_VehStandStillSts == false) &&...
              | (kmph_VehLgtSpd >- p_SHLA_VehSpdThd_kmph))) && ...
              | bool_ShftLvrAllwd]
          Reverse -> Neutral_tmp [order 1] : [bool_UnlockBtnPresd == true&& ...
              | (st_ShftLvrPstnTip == ShiftLvrPosnTipTyp.TIP_DOWN && ...
              | st_ShiftLvrPosn == ShiftLvrPosnTyp.SHL_R) ]
          Drive -> Neutral_tmp : [(st_ShftLvrPstnTip == ShiftLvrPosnTipTyp.TIP_UP && ...
              | st_ShiftLvrPosn == ShiftLvrPosnTyp.SHL_D) ]
          Neutral_tmp -> Reverse [order 1] : [after (p_SHLA_TiDlyShiftLvr_s ,sec) && ...
              | st_ShftLvrPstnTip == ShiftLvrPosnTipTyp.TIP_UP && ...
              | bool_UnlockBtnPresd == true && ...
              | kmph_VehLgtSpd < p_SHLA_VehSpdThd_kmph && ...
              | bool_ShftLvrAllwd]
          Neutral_tmp -> Drive [order 3] : [after (p_SHLA_TiDlyShiftLvr_s ,sec) && ...
              | st_ShftLvrPstnTip == ShiftLvrPosnTipTyp.TIP_DOWN && ...
              | kmph_VehLgtSpd > -p_SHLA_VehSpdThd_kmph && ...
              | bool_ShftLvrAllwd]
          (default) -> (junction 27)
          (junction 27) -> Driving.DRIVING.E_park_deactive.Shift_lever_logic.Neutral [order 3]
          (junction 27) -> Drive [order 1] : [st_ShftLvrPstnTip == ShiftLvrPosnTipTyp.TIP_DOWN]
      state Init
      (default) -> Driving.DRIVING.Init
      Driving.DRIVING.Init -> Driving.DRIVING.E_park_active [order 1] : [st_ShiftLvrPosn == ShiftLvrPosnTyp.SHL_P]
      Driving.DRIVING.Init -> E_park_deactive [order 2] : [st_ShiftLvrPosn == ShiftLvrPosnTyp.SHL_N]
      E_park_deactive -> Driving.DRIVING.E_park_active : [((st_PrkgLockBtn && ...
          | (abs(kmph_VehLgtSpd) < p_SHLA_LockPVehSpdThd_kmph)) || ...
          | (st_DrvDoorSt && ...
          | bool_BrkPedPrsd == false && ...
          | abs(kmph_VehLgtSpd) < p_SHLA_LockPVehSpdThd_kmph)) && ...
          | st_ShiftLvrPosn ~= ShiftLvrPosnTyp.SHL_P && ...
          | bool_ShftLvrAllwd]
      Driving.DRIVING.E_park_active -> E_park_deactive [order 1] : [bool_BrkPedPrsd && ...
          | (st_ShftLvrPstnTip == ShiftLvrPosnTipTyp.TIP_UP || ...
          | st_ShftLvrPstnTip == ShiftLvrPosnTipTyp.TIP_DOWN) && ...
          | st_ShiftLvrPosn == ShiftLvrPosnTyp.SHL_P]
  state Init
    en:
    bool_PrkgLock = true;
    st_ShiftLvrPosn = ShiftLvrPosnTyp.SHL_P;
  (default) -> Init
  E_park -> Drive_ready : [st_PtCoorrSts == VMMCoorrStsTyp.VMM_KeyOn || ...
      | st_PtCoorrSts == VMMCoorrStsTyp.VMM_DrvOn || ...
      | st_PtCoorrSts == VMMCoorrStsTyp.VMM_DrvOnOk || ...
      | st_PtCoorrSts == VMMCoorrStsTyp.VMM_Drv]
  Drive_ready -> Driving [order 1] : [st_PtCoorrSts == VMMCoorrStsTyp.VMM_Drv]
  Driving -> E_park : [st_PtCoorrSts != VMMCoorrStsTyp.VMM_Drv && ...
      | abs(kmph_VehLgtSpd) < p_SHLA_LockPVehSpdThd_kmph && ...
      | bool_ShftLvrAllwd]
  Drive_ready -> E_park [order 2] : [st_PtCoorrSts == VMMCoorrStsTyp.VMM_ShtDwn || ...
      | st_PtCoorrSts == VMMCoorrStsTyp.VMM_SafeMode]
  Init -> E_park : [st_EParkSt == PrkgLockStsTyp.PLS_PARKED || ...
      | st_EParkSt == PrkgLockStsTyp.PLS_UNPARKED]
  data: st_PtCoorrSts input double; bool_PrkgLock output boolean; st_ShiftLvrPosn output uint8; bool_BrkPedPrsd input double; st_PrkgLockBtn input double; st_ShftLvrPstnTip input double; kmph_VehLgtSpd input double; st_RecupLvl output uint8; TranEna local double; p_SHLA_VehSpdThd_kmph parameter double; p_SHLA_TiDlyShiftLvr_s parameter double; st_EParkSt input double; bool_ShftLvrAllwd input double; st_DrvDoorSt input double; bool_UnlockBtnPresd input double; bool_VehStandStillSts input double; p_SHLA_LockPVehSpdThd_kmph parameter double

== stateflow chart SHLA/Algo/EparkCtrl/Chart ==
  state Park
    state Parking
      en:
      st_PrkgLock=st_ParkReq;
    state Stalled
    state Parked
      en:
      st_PrkgLock=st_ParkReqOff;
      st_EparkSt=st_ParkLocked;
    state ParkFlt
      en:
      st_PrkgLock=st_ParkReqOff;
      st_EparkSt=st_ParkFlt;
    Park.Stalled -> ParkFlt [order 2] : [after(s_StalledDelyTime,sec)]
    Parking -> Parked [order 2] : [bool_PrkSnsr==bool_True]
    Parking -> Park.Stalled [order 1] : [st_PrkgLockSt==st_ParkStalled]
    (default) -> Parking
    Park.Stalled -> Parking [order 1] : [st_PrkgLockSt!=st_ParkStalled]
  state UnPark
    state UnParking
      en:
      st_PrkgLock=st_UnParkReq;
    state Stalled
    state UnParked
      en:
      st_PrkgLock=st_ParkReqOff;
      st_EparkSt=st_ParkUnlocked;
    state UnParkFlt
      en:
      st_PrkgLock=st_ParkReqOff;
      st_EparkSt=st_ParkFlt;
    UnPark.Stalled -> UnParkFlt [order 1] : [after(s_StalledDelyTime,sec)]
    UnParking -> UnParked [order 2] : [bool_DrvSensor==bool_True]
    UnParking -> UnPark.Stalled [order 1] : [st_PrkgLockSt==st_UnparkedStalled]
    (default) -> UnParking
    UnPark.Stalled -> UnParking [order 2] : [st_PrkgLockSt!=st_UnparkedStalled]
  Park -> UnPark : [bool_PrkgLock==bool_False]
  (default) -> Park
  UnPark -> Park : [bool_PrkgLock==bool_True]
  data: bool_PrkgLock input double; bool_DrvSensor input double; bool_PrkSnsr input double; st_PrkgLockSt input double; bool_True input double; bool_False input double; st_Parking input double; st_Parked input double; st_ParkStalled input double; st_Unparking input double; st_Unparked input double; st_UnparkedStalled input double; st_ParkLockUnknown input double; st_ParkReqOff input double; st_ParkReq input double; st_UnParkReq input double; st_ParkLocked input double; st_ParkFlt input double; st_ParkUnlocked input double; st_EparkSt output uint8; st_PrkgLock output uint8; s_StalledDelyTime input double

== stateflow chart SHLA/Algo/Algo/Vehicle_StandStill_Status/Chart_VehStandStill ==
  state VehStandStill
    en:
    bool_VehStandStillSts = true;
  state VehMove
    en:
    bool_VehStandStillSts = false;
  state VehStandStill_Delay
  (default) -> VehStandStill
  VehStandStill -> VehMove : [rpm_MotCtlrActRev>=pMCI_rpm_VehMoveSpdThrsh_C]
  VehStandStill_Delay -> VehStandStill [order 2] : [rpm_MotCtlrActRev<pMCI_rpm_VehStdStlSpdThrsh_C&& ...
      | after(pMCI_s_VehStdStlDly_C, sec)]
  VehMove -> VehStandStill_Delay : [rpm_MotCtlrActRev<pMCI_rpm_VehStdStlSpdThrsh_C]
  VehStandStill_Delay -> VehMove [order 1] : [rpm_MotCtlrActRev>=pMCI_rpm_VehMoveSpdThrsh_C]
  data: rpm_MotCtlrActRev input double; bool_VehStandStillSts output boolean; pMCI_rpm_VehStdStlSpdThrsh_C parameter double; pMCI_s_VehStdStlDly_C parameter double; pMCI_rpm_VehMoveSpdThrsh_C parameter double
